simulink model "roll_loop"  (R2016b)
settings: Solver=VariableStepAuto  StartTime=0.0  StopTime=10.0  RelTol=1e-3
undefined symbols (not defined in the file): a_phi1, a_phi2, k_d_phi, k_p_phi
settings Model: Creator=geun2  LastModifiedBy=geun2

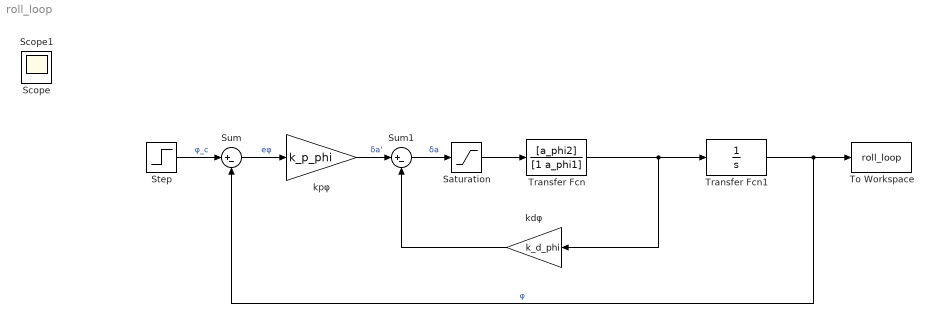
== system roll_loop ==
  Saturation : Saturate  UpperLimit=45*pi/180  LowerLimit=-45*pi/180
  Step : Step  After=15*pi/180  SampleTime=0
  Sum : Sum  Inputs=|+-
  Sum1 : Sum  Inputs=|+-
  To Workspace : ToWorkspace  VariableName=roll_loop  SaveFormat=Timeseries  SampleTime=-1
  Transfer Fcn : TransferFcn  Numerator=[a_phi2]  Denominator=[1 a_phi1]
  Transfer Fcn1 : TransferFcn  Denominator=[1 0]
  kdφ : Gain  Gain=k_d_phi
  kpφ : Gain  Gain=k_p_phi
  Scope : Scope
  Scope1 : Scope
  wires:
  Sum/1 -> kpφ/1  "eφ"
  kpφ/1 -> Sum1/1  "δa'"
  Sum1/1 -> Saturation/1  "δa"
  Transfer Fcn/1 -> Transfer Fcn1/1, kdφ/1
  Transfer Fcn1/1 -> Sum/2, To Workspace/1  "φ"
  kdφ/1 -> Sum1/2
  Step/1 -> Sum/1  "φ_c"
  Saturation/1 -> Transfer Fcn/1
